simulink model "MaquinaDeEstados_Driverless"  (R2019b)
settings: Solver=VariableStepAuto  StartTime=0.0  StopTime=10.0  RelTol=1e-3
settings Model: Creator=bujan  LastModifiedBy=PABLO
settings DebuggingCC: UnderSpecifiedDimensionMsg=warning
settings ConfigComp: PLC_TargetIDE=plcopen

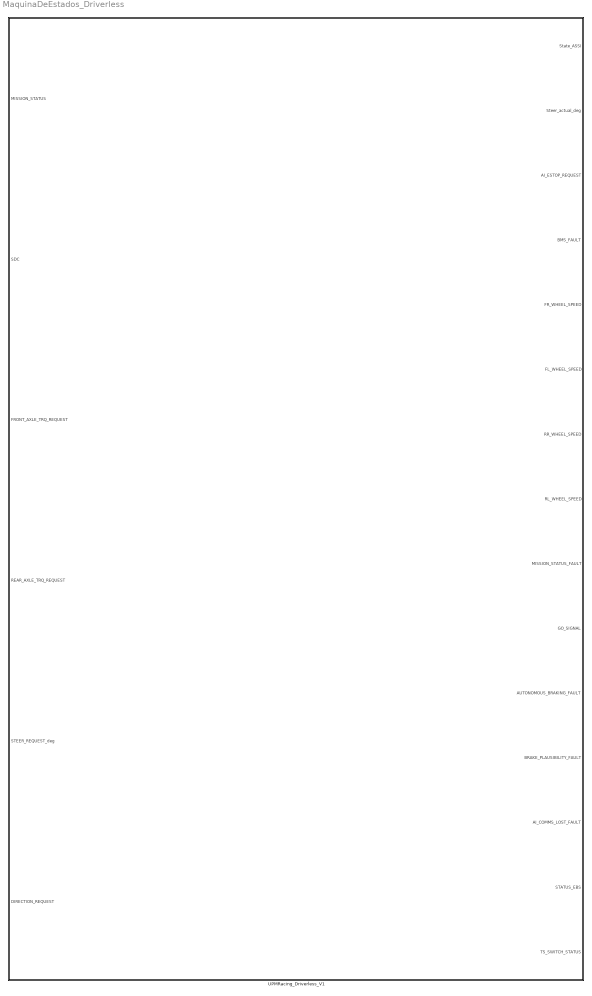
== system MaquinaDeEstados_Driverless ==
  "UPMRacing_Driverless_V1 " : Stateflow chart  TreatAsAtomicUnit=on

== stateflow chart MaquinaDeEstados_Driverless/UPMRacing_Driverless_V1  ==
  state Main [parallel]
    settings: executionOrder=1
    state AS_READY
      entry:
      State_ASSI=2
    state INTERMIDIATE
      entry:
      State_ASSI=2
    state AS_DRIVING
      entry:
      State_ASSI=3
    state EMERGENCY_BRAKE
      entry:
      State_ASSI=4
    state AS_FINISHED
      entry:
      State_ASSI=5
    state EMERGENCY_BRAKE_COMPLETED
      entry:
      State_ASSI=4
    state AS_OFF
      entry:
      State_ASSI = 1
    INTERMIDIATE -> AS_READY [order 3] : [FRONT_AXLE_TRQ_REQUEST ~= 0 ||...
        | REAR_AXLE_TRQ_REQUEST  ~= 0 ||...
        | STEER_REQUEST_deg  ~= 0 ||...
        | Steer_actual_deg >= 5  ||...
        | DIRECTION_REQUEST ~= 0]
    INTERMIDIATE -> AS_DRIVING [order 1] : [GO_SIGNAL == 1]
    AS_READY -> INTERMIDIATE [order 3] : [after(5,sec) &...
        | FRONT_AXLE_TRQ_REQUEST == 0 &...
        | REAR_AXLE_TRQ_REQUEST  == 0 &...
        | STEER_REQUEST_deg  == 0 &...
        | Steer_actual_deg < 5  &...
        | DIRECTION_REQUEST == 0 &...
        | GO_SIGNAL == 0]
    AS_READY -> EMERGENCY_BRAKE [order 2] : [SDC==0]
    AS_DRIVING -> EMERGENCY_BRAKE [order 2] : [SDC==0 ||...
        | AS_SWITCH_STATUS == 0 ||...
        | GO_SIGNAL == 0 ||...
        | MISSION_STATUS_FAULT == 1 ||...
        | AUTONOMOUS_BRAKING_FAULT == 1 || ...
        | BRAKE_PLAUSIBILITY_FAULT == 1 ||...
        | AI_ESTOP_REQUEST == 1 ||...
        | AI_COMMS_LOST_FAULT == 1 ||...
        | BMS_FAULT == 1 ||...
        | STATUS_EBS == 1]
    AS_OFF -> AS_READY : [AS_SWITCH_STATUS == 1 &...
        | TS_SWITCH_STATUS == 1 &...
        | STATUS_EBS == 2 &...
        | MISSION_STATUS == 1]
    AS_READY -> AS_OFF [order 1] : [AS_SWITCH_STATUS == 0]
    INTERMIDIATE -> EMERGENCY_BRAKE [order 2] : [SDC==0]
    AS_DRIVING -> AS_FINISHED [order 1] : [MISSION_STATUS == 3 &...
        | FR_WHEEL_SPEED<10 &...
        | FL_WHEEL_SPEED<10 &...
        | RR_WHEEL_SPEED<10 &...
        | RL_WHEEL_SPEED<10]
    AS_FINISHED -> EMERGENCY_BRAKE [order 2] : [SDC==0]
    AS_FINISHED -> AS_OFF [order 1] : [AS_SWITCH_STATUS == 0]
    EMERGENCY_BRAKE -> EMERGENCY_BRAKE_COMPLETED : [after(15,sec)]
    EMERGENCY_BRAKE_COMPLETED -> AS_OFF : [AS_SWITCH_STATUS == 0]
    (default) -> AS_OFF
  data: MISSION_STATUS input uint8; State_ASSI output uint8 size=1; SDC input boolean; FRONT_AXLE_TRQ_REQUEST input uint16; REAR_AXLE_TRQ_REQUEST input uint16; STEER_REQUEST_deg input fixdt(1,16,2^0,0); Steer_actual_deg output int8 size=1; DIRECTION_REQUEST input boolean; AI_ESTOP_REQUEST output boolean size=1; BMS_FAULT output boolean size=1; FR_WHEEL_SPEED output uint16 size=1; FL_WHEEL_SPEED output uint16 size=1; RR_WHEEL_SPEED output uint16 size=1; RL_WHEEL_SPEED output uint16 size=1; MISSION_STATUS_FAULT output boolean size=1; GO_SIGNAL output boolean size=1; AUTONOMOUS_BRAKING_FAULT output boolean size=1; BRAKE_PLAUSIBILITY_FAULT output boolean size=1; AI_COMMS_LOST_FAULT output boolean size=1; STATUS_EBS output uint8 size=1; AS_SWITCH_STATUS local boolean size=1; TS_SWITCH_STATUS output boolean size=1
